simulink library "sm_trackV_lib_belt_underc_idlerArm_i2u0l3"  (R2026a)
settings: Solver=VariableStepAuto
undefined symbols (not defined in the file): A, Fixed, L1, L2, L3, Right, S, Trac, X, Y, Z
libraries: sm_lib x11, sm_trackV_lib_belt_underc_elem x9, nesl_utility x7, fl_lib x2, sm_trackV_lib_frame_idlerArm_i2u0l3 x1
(part 2 of 2)

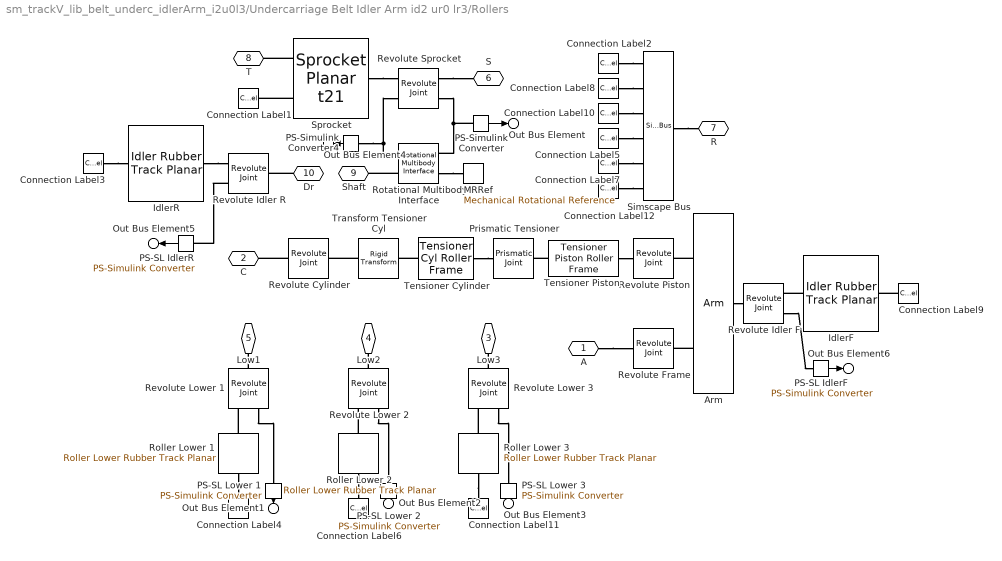
== system sm_trackV_lib_belt_underc_idlerArm_i2u0l3/Undercarriage Belt Idler Arm id2 ur0 lr3/Rollers ==
  Arm : sm_trackV_lib_belt_underc_elem/Arm  arm_idlerc=arm_idlerc  arm_tens_x=arm_tens_x  arm_tens_y=arm_tens_y  arm_wid=arm_wid  arm_thk=arm_thk  arm_rho=arm_rho  arm_clr=arm_clr  arm_opc=arm_opc
  Connection Label1 : ConnectionLabel  Label=S
  Connection Label10 : ConnectionLabel  Label=A
  Connection Label11 : ConnectionLabel  Label=L3
  Connection Label12 : ConnectionLabel  Label=L3
  Connection Label2 : ConnectionLabel  Label=S
  Connection Label3 : ConnectionLabel  Label=X
  Connection Label4 : ConnectionLabel  Label=L1
  Connection Label5 : ConnectionLabel  Label=L1
  Connection Label6 : ConnectionLabel  Label=L2
  Connection Label7 : ConnectionLabel  Label=L2
  Connection Label8 : ConnectionLabel  Label=X
  Connection Label9 : ConnectionLabel  Label=A
  IdlerF : sm_trackV_lib_belt_underc_elem/Idler Rubber Track Planar  idler_rad=idlerF_rad  idler_len=idlerF_len  wheel_clr=idlerF_wheel_clr  rim_rad=IdlerF_rim_rad  rim_hub_rad=idlerF_rim_hub_rad  rim_xc=idlerF_rim_xc  idler_rho=idlerF_rho  idler_opc=idlerF_opc  idler_clr=idlerF_clr  idler_axle_rad=idlerF_axle_rad  idler_axle_len=idlerF_axle_len  idler_axle_rho=idlerF_axle_rho  idler_axle_opc=idlerF_axle_opc  idler_axle_clr=idlerF_axle_clr  idler_contgeo_clr=idlerF_contgeo_clr  idler_contgeo_opc=idlerF_contgeo_opc
  IdlerR : sm_trackV_lib_belt_underc_elem/Idler Rubber Track Planar  idler_rad=idlerR_rad  idler_len=idlerR_len  wheel_clr=idlerR_wheel_clr  rim_rad=idlerR_rim_rad  rim_hub_rad=idlerR_rim_hub_rad  rim_xc=idlerR_rim_xc  idler_rho=idlerR_rho  idler_opc=idlerR_opc  idler_clr=idlerR_clr  idler_axle_rad=idlerR_axle_rad  idler_axle_len=idlerR_axle_len  idler_axle_rho=idlerR_axle_rho  idler_axle_opc=idlerR_axle_opc  idler_axle_clr=idlerR_axle_clr  idler_contgeo_clr=idlerR_contgeo_clr  idler_contgeo_opc=idlerR_contgeo_opc
  MRRef : fl_lib/Mechanical/Rotational Elements/Mechanical Rotational Reference
  PS-SL IdlerF : nesl_utility/PS-Simulink Converter  PhysicalDomain=network_engine_domain  SubClassName=ps_output  LeftPortType=input  RightPortType=output  PseudoPeriodic=off  Frequencies=[]  VectorFormat=inherit  Unit=inherit  AffineConversion=off
  PS-SL IdlerR : nesl_utility/PS-Simulink Converter  PhysicalDomain=network_engine_domain  SubClassName=ps_output  LeftPortType=input  RightPortType=output  PseudoPeriodic=off  Frequencies=[]  VectorFormat=inherit  Unit=inherit  AffineConversion=off
  PS-SL Lower 1 : nesl_utility/PS-Simulink Converter  PhysicalDomain=network_engine_domain  SubClassName=ps_output  LeftPortType=input  RightPortType=output  PseudoPeriodic=off  Frequencies=[]  VectorFormat=inherit  Unit=inherit  AffineConversion=off
  PS-SL Lower 2 : nesl_utility/PS-Simulink Converter  PhysicalDomain=network_engine_domain  SubClassName=ps_output  LeftPortType=input  RightPortType=output  PseudoPeriodic=off  Frequencies=[]  VectorFormat=inherit  Unit=inherit  AffineConversion=off
  PS-SL Lower 3 : nesl_utility/PS-Simulink Converter  PhysicalDomain=network_engine_domain  SubClassName=ps_output  LeftPortType=input  RightPortType=output  PseudoPeriodic=off  Frequencies=[]  VectorFormat=inherit  Unit=inherit  AffineConversion=off
  PS-Simulink Converter : nesl_utility/PS-Simulink Converter  PhysicalDomain=network_engine_domain  SubClassName=ps_output  LeftPortType=input  RightPortType=output  PseudoPeriodic=off  Frequencies=[]  VectorFormat=inherit  Unit=inherit  AffineConversion=off
  PS-Simulink Converter4 : nesl_utility/PS-Simulink Converter  PhysicalDomain=network_engine_domain  SubClassName=ps_output  LeftPortType=input  RightPortType=output  PseudoPeriodic=off  Frequencies=[]  VectorFormat=inherit  Unit=inherit  AffineConversion=off
  Prismatic Tensioner : sm_lib/Joints/Prismatic Joint  JointMode=Normal  CompositeWrenchDir=FollowerOnBase  CompositeWrenchFrame=BaseFrame  SenseConstraintForce=off  SenseConstraintTorque=off  SenseTotalForce=off  SenseTotalTorque=off  PositionTargetSpecify=on  PositionTargetPriority=High  PositionTargetValue=tensioner_x0  PositionTargetValueUnits=m  VelocityTargetSpecify=off  VelocityTargetPriority=High  VelocityTargetValue=0  VelocityTargetValueUnits=m/s  EquilibriumPosition=tensioner_eqpos  EquilibriumPositionUnits=m  SpringStiffness=tensioner_k  SpringStiffnessUnits=N/m  DampingCoefficient=tensioner_b  DampingCoefficientUnits=N/(m/s)  LowerLimitSpecify=off  LowerLimitBound=-1  LowerLimitBoundUnits=m  LowerLimitStiffness=1e6  LowerLimitStiffnessUnits=N/m  LowerLimitDamping=1e3  LowerLimitDampingUnits=N/(m/s)  LowerLimitTransitionRegionWidth=1e-4  LowerLimitTransitionRegionWidthUnits=m  UpperLimitSpecify=off  UpperLimitBound=1  UpperLimitBoundUnits=m  UpperLimitStiffness=1e6  UpperLimitStiffnessUnits=N/m  UpperLimitDamping=1e3  UpperLimitDampingUnits=N/(m/s)  UpperLimitTransitionRegionWidth=1e-4  UpperLimitTransitionRegionWidthUnits=m  TorqueActuationMode=NoTorque  MotionActuationMode=ComputedMotion  SensePosition=off  SenseVelocity=off  SenseAcceleration=off  SenseTorqueForce=off  SenseLowerLimitTorqueForce=off  SenseUpperLimitTorqueForce=off
  Revolute Cylinder : sm_lib/Joints/Revolute Joint  JointMode=Normal  CompositeWrenchDir=FollowerOnBase  CompositeWrenchFrame=BaseFrame  SenseConstraintForce=off  SenseConstraintTorque=off  SenseTotalForce=off  SenseTotalTorque=off  PositionTargetSpecify=on  PositionTargetPriority=Low  PositionTargetValue=0  PositionTargetValueUnits=deg  VelocityTargetSpecify=off  VelocityTargetPriority=High  VelocityTargetValue=0  VelocityTargetValueUnits=deg/s  EquilibriumPosition=0  EquilibriumPositionUnits=deg  SpringStiffness=0  SpringStiffnessUnits=N*m/deg  DampingCoefficient=0  DampingCoefficientUnits=N*m/(deg/s)  LowerLimitSpecify=off  LowerLimitBound=-90  LowerLimitBoundUnits=deg  LowerLimitStiffness=1e4  LowerLimitStiffnessUnits=N*m/deg  LowerLimitDamping=10  LowerLimitDampingUnits=N*m/(deg/s)  LowerLimitTransitionRegionWidth=0.1  LowerLimitTransitionRegionWidthUnits=deg  UpperLimitSpecify=off  UpperLimitBound=90  UpperLimitBoundUnits=deg  UpperLimitStiffness=1e4  UpperLimitStiffnessUnits=N*m/deg  UpperLimitDamping=10  UpperLimitDampingUnits=N*m/(deg/s)  UpperLimitTransitionRegionWidth=0.1  UpperLimitTransitionRegionWidthUnits=deg  TorqueActuationMode=NoTorque  MotionActuationMode=ComputedMotion  SensePosition=off  SenseVelocity=off  SenseAcceleration=off  SenseTorqueForce=off  SenseLowerLimitTorqueForce=off  SenseUpperLimitTorqueForce=off
  Revolute Frame : sm_lib/Joints/Revolute Joint  JointMode=Normal  CompositeWrenchDir=FollowerOnBase  CompositeWrenchFrame=BaseFrame  SenseConstraintForce=off  SenseConstraintTorque=off  SenseTotalForce=off  SenseTotalTorque=off  PositionTargetSpecify=off  PositionTargetPriority=Low  PositionTargetValue=0  PositionTargetValueUnits=deg  VelocityTargetSpecify=off  VelocityTargetPriority=High  VelocityTargetValue=0  VelocityTargetValueUnits=deg/s  EquilibriumPosition=0  EquilibriumPositionUnits=rad  SpringStiffness=0  SpringStiffnessUnits=N*m/rad  DampingCoefficient=0  DampingCoefficientUnits=N*m/(rad/s)  LowerLimitSpecify=off  LowerLimitBound=-90  LowerLimitBoundUnits=deg  LowerLimitStiffness=1e4  LowerLimitStiffnessUnits=N*m/deg  LowerLimitDamping=10  LowerLimitDampingUnits=N*m/(deg/s)  LowerLimitTransitionRegionWidth=0.1  LowerLimitTransitionRegionWidthUnits=deg  UpperLimitSpecify=off  UpperLimitBound=90  UpperLimitBoundUnits=deg  UpperLimitStiffness=1e4  UpperLimitStiffnessUnits=N*m/deg  UpperLimitDamping=10  UpperLimitDampingUnits=N*m/(deg/s)  UpperLimitTransitionRegionWidth=0.1  UpperLimitTransitionRegionWidthUnits=deg  TorqueActuationMode=NoTorque  MotionActuationMode=ComputedMotion  SensePosition=off  SenseVelocity=off  SenseAcceleration=off  SenseTorqueForce=off  SenseLowerLimitTorqueForce=off  SenseUpperLimitTorqueForce=off
  Revolute Idler F : sm_lib/Joints/Revolute Joint  JointMode=Normal  CompositeWrenchDir=FollowerOnBase  CompositeWrenchFrame=BaseFrame  SenseConstraintForce=on  SenseConstraintTorque=off  SenseTotalForce=off  SenseTotalTorque=off  PositionTargetSpecify=off  PositionTargetPriority=Low  PositionTargetValue=0  PositionTargetValueUnits=deg  VelocityTargetSpecify=off  VelocityTargetPriority=High  VelocityTargetValue=0  VelocityTargetValueUnits=deg/s  EquilibriumPosition=0  EquilibriumPositionUnits=rad  SpringStiffness=0  SpringStiffnessUnits=N*m/rad  DampingCoefficient=0  DampingCoefficientUnits=N*m/(rad/s)  LowerLimitSpecify=off  LowerLimitBound=-90  LowerLimitBoundUnits=deg  LowerLimitStiffness=1e4  LowerLimitStiffnessUnits=N*m/deg  LowerLimitDamping=10  LowerLimitDampingUnits=N*m/(deg/s)  LowerLimitTransitionRegionWidth=0.1  LowerLimitTransitionRegionWidthUnits=deg  UpperLimitSpecify=off  UpperLimitBound=90  UpperLimitBoundUnits=deg  UpperLimitStiffness=1e4  UpperLimitStiffnessUnits=N*m/deg  UpperLimitDamping=10  UpperLimitDampingUnits=N*m/(deg/s)  UpperLimitTransitionRegionWidth=0.1  UpperLimitTransitionRegionWidthUnits=deg  TorqueActuationMode=NoTorque  MotionActuationMode=ComputedMotion  SensePosition=off  SenseVelocity=off  SenseAcceleration=off  SenseTorqueForce=off  SenseLowerLimitTorqueForce=off  SenseUpperLimitTorqueForce=off
  Revolute Idler R : sm_lib/Joints/Revolute Joint  JointMode=Normal  CompositeWrenchDir=FollowerOnBase  CompositeWrenchFrame=BaseFrame  SenseConstraintForce=on  SenseConstraintTorque=off  SenseTotalForce=off  SenseTotalTorque=off  PositionTargetSpecify=off  PositionTargetPriority=Low  PositionTargetValue=0  PositionTargetValueUnits=deg  VelocityTargetSpecify=off  VelocityTargetPriority=High  VelocityTargetValue=0  VelocityTargetValueUnits=deg/s  EquilibriumPosition=0  EquilibriumPositionUnits=rad  SpringStiffness=0  SpringStiffnessUnits=N*m/rad  DampingCoefficient=0  DampingCoefficientUnits=N*m/(rad/s)  LowerLimitSpecify=off  LowerLimitBound=-90  LowerLimitBoundUnits=deg  LowerLimitStiffness=1e4  LowerLimitStiffnessUnits=N*m/deg  LowerLimitDamping=10  LowerLimitDampingUnits=N*m/(deg/s)  LowerLimitTransitionRegionWidth=0.1  LowerLimitTransitionRegionWidthUnits=deg  UpperLimitSpecify=off  UpperLimitBound=90  UpperLimitBoundUnits=deg  UpperLimitStiffness=1e4  UpperLimitStiffnessUnits=N*m/deg  UpperLimitDamping=10  UpperLimitDampingUnits=N*m/(deg/s)  UpperLimitTransitionRegionWidth=0.1  UpperLimitTransitionRegionWidthUnits=deg  TorqueActuationMode=NoTorque  MotionActuationMode=ComputedMotion  SensePosition=off  SenseVelocity=off  SenseAcceleration=off  SenseTorqueForce=off  SenseLowerLimitTorqueForce=off  SenseUpperLimitTorqueForce=off
  Revolute Lower 1 : sm_lib/Joints/Revolute Joint  JointMode=Normal  CompositeWrenchDir=FollowerOnBase  CompositeWrenchFrame=BaseFrame  SenseConstraintForce=on  SenseConstraintTorque=off  SenseTotalForce=off  SenseTotalTorque=off  PositionTargetSpecify=off  PositionTargetPriority=Low  PositionTargetValue=0  PositionTargetValueUnits=deg  VelocityTargetSpecify=off  VelocityTargetPriority=High  VelocityTargetValue=0  VelocityTargetValueUnits=deg/s  EquilibriumPosition=0  EquilibriumPositionUnits=rad  SpringStiffness=0  SpringStiffnessUnits=N*m/rad  DampingCoefficient=0  DampingCoefficientUnits=N*m/(rad/s)  LowerLimitSpecify=off  LowerLimitBound=-90  LowerLimitBoundUnits=deg  LowerLimitStiffness=1e4  LowerLimitStiffnessUnits=N*m/deg  LowerLimitDamping=10  LowerLimitDampingUnits=N*m/(deg/s)  LowerLimitTransitionRegionWidth=0.1  LowerLimitTransitionRegionWidthUnits=deg  UpperLimitSpecify=off  UpperLimitBound=90  UpperLimitBoundUnits=deg  UpperLimitStiffness=1e4  UpperLimitStiffnessUnits=N*m/deg  UpperLimitDamping=10  UpperLimitDampingUnits=N*m/(deg/s)  UpperLimitTransitionRegionWidth=0.1  UpperLimitTransitionRegionWidthUnits=deg  TorqueActuationMode=NoTorque  MotionActuationMode=ComputedMotion  SensePosition=off  SenseVelocity=off  SenseAcceleration=off  SenseTorqueForce=off  SenseLowerLimitTorqueForce=off  SenseUpperLimitTorqueForce=off
  Revolute Lower 2 : sm_lib/Joints/Revolute Joint  JointMode=Normal  CompositeWrenchDir=FollowerOnBase  CompositeWrenchFrame=BaseFrame  SenseConstraintForce=on  SenseConstraintTorque=off  SenseTotalForce=off  SenseTotalTorque=off  PositionTargetSpecify=off  PositionTargetPriority=Low  PositionTargetValue=0  PositionTargetValueUnits=deg  VelocityTargetSpecify=off  VelocityTargetPriority=High  VelocityTargetValue=0  VelocityTargetValueUnits=deg/s  EquilibriumPosition=0  EquilibriumPositionUnits=rad  SpringStiffness=0  SpringStiffnessUnits=N*m/rad  DampingCoefficient=0  DampingCoefficientUnits=N*m/(rad/s)  LowerLimitSpecify=off  LowerLimitBound=-90  LowerLimitBoundUnits=deg  LowerLimitStiffness=1e4  LowerLimitStiffnessUnits=N*m/deg  LowerLimitDamping=10  LowerLimitDampingUnits=N*m/(deg/s)  LowerLimitTransitionRegionWidth=0.1  LowerLimitTransitionRegionWidthUnits=deg  UpperLimitSpecify=off  UpperLimitBound=90  UpperLimitBoundUnits=deg  UpperLimitStiffness=1e4  UpperLimitStiffnessUnits=N*m/deg  UpperLimitDamping=10  UpperLimitDampingUnits=N*m/(deg/s)  UpperLimitTransitionRegionWidth=0.1  UpperLimitTransitionRegionWidthUnits=deg  TorqueActuationMode=NoTorque  MotionActuationMode=ComputedMotion  SensePosition=off  SenseVelocity=off  SenseAcceleration=off  SenseTorqueForce=off  SenseLowerLimitTorqueForce=off  SenseUpperLimitTorqueForce=off
  Revolute Lower 3 : sm_lib/Joints/Revolute Joint  JointMode=Normal  CompositeWrenchDir=FollowerOnBase  CompositeWrenchFrame=BaseFrame  SenseConstraintForce=on  SenseConstraintTorque=off  SenseTotalForce=off  SenseTotalTorque=off  PositionTargetSpecify=off  PositionTargetPriority=Low  PositionTargetValue=0  PositionTargetValueUnits=deg  VelocityTargetSpecify=off  VelocityTargetPriority=High  VelocityTargetValue=0  VelocityTargetValueUnits=deg/s  EquilibriumPosition=0  EquilibriumPositionUnits=rad  SpringStiffness=0  SpringStiffnessUnits=N*m/rad  DampingCoefficient=0  DampingCoefficientUnits=N*m/(rad/s)  LowerLimitSpecify=off  LowerLimitBound=-90  LowerLimitBoundUnits=deg  LowerLimitStiffness=1e4  LowerLimitStiffnessUnits=N*m/deg  LowerLimitDamping=10  LowerLimitDampingUnits=N*m/(deg/s)  LowerLimitTransitionRegionWidth=0.1  LowerLimitTransitionRegionWidthUnits=deg  UpperLimitSpecify=off  UpperLimitBound=90  UpperLimitBoundUnits=deg  UpperLimitStiffness=1e4  UpperLimitStiffnessUnits=N*m/deg  UpperLimitDamping=10  UpperLimitDampingUnits=N*m/(deg/s)  UpperLimitTransitionRegionWidth=0.1  UpperLimitTransitionRegionWidthUnits=deg  TorqueActuationMode=NoTorque  MotionActuationMode=ComputedMotion  SensePosition=off  SenseVelocity=off  SenseAcceleration=off  SenseTorqueForce=off  SenseLowerLimitTorqueForce=off  SenseUpperLimitTorqueForce=off
  Revolute Piston : sm_lib/Joints/Revolute Joint  JointMode=Normal  CompositeWrenchDir=FollowerOnBase  CompositeWrenchFrame=BaseFrame  SenseConstraintForce=off  SenseConstraintTorque=off  SenseTotalForce=off  SenseTotalTorque=off  PositionTargetSpecify=off  PositionTargetPriority=Low  PositionTargetValue=0  PositionTargetValueUnits=deg  VelocityTargetSpecify=off  VelocityTargetPriority=High  VelocityTargetValue=0  VelocityTargetValueUnits=deg/s  EquilibriumPosition=0  EquilibriumPositionUnits=rad  SpringStiffness=0  SpringStiffnessUnits=N*m/rad  DampingCoefficient=0  DampingCoefficientUnits=N*m/(rad/s)  LowerLimitSpecify=off  LowerLimitBound=-90  LowerLimitBoundUnits=deg  LowerLimitStiffness=1e4  LowerLimitStiffnessUnits=N*m/deg  LowerLimitDamping=10  LowerLimitDampingUnits=N*m/(deg/s)  LowerLimitTransitionRegionWidth=0.1  LowerLimitTransitionRegionWidthUnits=deg  UpperLimitSpecify=off  UpperLimitBound=90  UpperLimitBoundUnits=deg  UpperLimitStiffness=1e4  UpperLimitStiffnessUnits=N*m/deg  UpperLimitDamping=10  UpperLimitDampingUnits=N*m/(deg/s)  UpperLimitTransitionRegionWidth=0.1  UpperLimitTransitionRegionWidthUnits=deg  TorqueActuationMode=NoTorque  MotionActuationMode=ComputedMotion  SensePosition=off  SenseVelocity=off  SenseAcceleration=off  SenseTorqueForce=off  SenseLowerLimitTorqueForce=off  SenseUpperLimitTorqueForce=off
  Revolute Sprocket : sm_lib/Joints/Revolute Joint  JointMode=Normal  CompositeWrenchDir=FollowerOnBase  CompositeWrenchFrame=BaseFrame  SenseConstraintForce=off  SenseConstraintTorque=off  SenseTotalForce=off  SenseTotalTorque=off  PositionTargetSpecify=off  PositionTargetPriority=Low  PositionTargetValue=0  PositionTargetValueUnits=deg  VelocityTargetSpecify=off  VelocityTargetPriority=High  VelocityTargetValue=0  VelocityTargetValueUnits=deg/s  EquilibriumPosition=0  EquilibriumPositionUnits=rad  SpringStiffness=0  SpringStiffnessUnits=N*m/rad  DampingCoefficient=0  DampingCoefficientUnits=N*m/(rad/s)  LowerLimitSpecify=off  LowerLimitBound=-90  LowerLimitBoundUnits=deg  LowerLimitStiffness=1e4  LowerLimitStiffnessUnits=N*m/deg  LowerLimitDamping=10  LowerLimitDampingUnits=N*m/(deg/s)  LowerLimitTransitionRegionWidth=0.1  LowerLimitTransitionRegionWidthUnits=deg  UpperLimitSpecify=off  UpperLimitBound=90  UpperLimitBoundUnits=deg  UpperLimitStiffness=1e4  UpperLimitStiffnessUnits=N*m/deg  UpperLimitDamping=10  UpperLimitDampingUnits=N*m/(deg/s)  UpperLimitTransitionRegionWidth=0.1  UpperLimitTransitionRegionWidthUnits=deg  TorqueActuationMode=InputTorque  MotionActuationMode=ComputedMotion  SensePosition=off  SenseVelocity=on  SenseAcceleration=off  SenseTorqueForce=off  SenseLowerLimitTorqueForce=off  SenseUpperLimitTorqueForce=off
  Roller Lower 1 : sm_trackV_lib_belt_underc_elem/Roller Lower Rubber Track Planar  roller_lower_rad=roller_lower_rad  roller_lower_len=roller_lower_len  roller_lower_rho=roller_lower_rho  roller_lower_clr=roller_lower_clr  roller_lower_opc=roller_lower_opc  roller_lower_rim_thk=roller_lower_rim_thk  roller_lower_rim_len=roller_lower_rim_len  roller_lower_axle_rad=roller_lower_axle_rad  roller_lower_axle_len=roller_lower_axle_len  roller_lower_axle_rho=roller_lower_axle_rho  roller_lower_axle_opc=roller_lower_axle_opc  roller_lower_axle_clr=roller_lower_axle_clr  roller_lower_contgeo_clr=roller_lower_contgeo_clr  roller_lower_contgeo_opc=roller_lower_contgeo_opc
  Roller Lower 2 : sm_trackV_lib_belt_underc_elem/Roller Lower Rubber Track Planar  roller_lower_rad=roller_lower_rad  roller_lower_len=roller_lower_len  roller_lower_rho=roller_lower_rho  roller_lower_clr=roller_lower_clr  roller_lower_opc=roller_lower_opc  roller_lower_rim_thk=roller_lower_rim_thk  roller_lower_rim_len=roller_lower_rim_len  roller_lower_axle_rad=roller_lower_axle_rad  roller_lower_axle_len=roller_lower_axle_len  roller_lower_axle_rho=roller_lower_axle_rho  roller_lower_axle_opc=roller_lower_axle_opc  roller_lower_axle_clr=roller_lower_axle_clr  roller_lower_contgeo_clr=roller_lower_contgeo_clr  roller_lower_contgeo_opc=roller_lower_contgeo_opc
  Roller Lower 3 : sm_trackV_lib_belt_underc_elem/Roller Lower Rubber Track Planar  roller_lower_rad=roller_lower_rad  roller_lower_len=roller_lower_len  roller_lower_rho=roller_lower_rho  roller_lower_clr=roller_lower_clr  roller_lower_opc=roller_lower_opc  roller_lower_rim_thk=roller_lower_rim_thk  roller_lower_rim_len=roller_lower_rim_len  roller_lower_axle_rad=roller_lower_axle_rad  roller_lower_axle_len=roller_lower_axle_len  roller_lower_axle_rho=roller_lower_axle_rho  roller_lower_axle_opc=roller_lower_axle_opc  roller_lower_axle_clr=roller_lower_axle_clr  roller_lower_contgeo_clr=roller_lower_contgeo_clr  roller_lower_contgeo_opc=roller_lower_contgeo_opc
  Rotational Multibody Interface : fl_lib/Mechanical/Multibody Interfaces/Rotational Multibody Interface
  Simscape Bus : SimscapeBus  HierarchyStrings=S;X;A;L1;L2;L3
  Sprocket : sm_trackV_lib_belt_underc_elem/Sprocket Planar t21  sprk_wid_roll=sprk_wid_roll  sprk_rad_roll=sprk_rad_roll  sprk_opc=sprk_opc  sprk_clr=sprk_clr  sprk_rad_pitch=sprk_rad_pitch  sprk_spoke_rad=sprk_spoke_rad  sprk_spoke_len=sprk_spoke_len  sprk_spoke_num=sprk_spoke_num  sprk_spoke_clr=sprk_clr  sprk_spoke_opc=sprk_opc  rim_spoke_xc=sprk_rim_spoke_xc  rim_thk=sprk_rim_thk  rim_ir=sprk_rim_ir  sprk_contgeo_roller_clr=sprk_contgeo_roller_clr  sprk_contgeo_roller_opc=sprk_contgeo_roller_opc  sprk_contgeo_spoke_clr=sprk_contgeo_spoke_clr  sprk_contgeo_spoke_opc=sprk_contgeo_spoke_opc
  Tensioner Cylinder : sm_trackV_lib_belt_underc_elem/Tensioner Cyl Roller Frame  cyl_rad=tensioner_cyl_rad  cyl_len=tensioner_cyl_len  cyl_rho=tensioner_cyl_rho  cyl_clr=tensioner_cyl_clr  cyl_opc=tensioner_cyl_opc
  Tensioner Piston : sm_trackV_lib_belt_underc_elem/Tensioner Piston Roller Frame  pist_rad=tensioner_pist_rad  pist_len=pist_len  pist_rho=tensioner_pist_rho  pist_clr=tensioner_pist_clr  pist_opc=tensioner_pist_opc  br_height=tensioner_br_height  br_length=brk_len  br_width=tensioner_br_width  br_rho=tensioner_br_rho  br_thk=brk_thk  br_clr=tensioner_br_clr  br_opc=tensioner_br_opc
  Transform Tensioner Cyl : sm_lib/Frames and Transforms/Rigid Transform  RotationMethod=AlignedAxes  FollAlignAxisA=+Z  BaseAlignAxisA=+X  FollAlignAxisB=+X  BaseAlignAxisB=+Y  RotationStandardAxis=+Y  RotationAngle=90  RotationAngleUnits=deg  RotationArbitraryAxis=[0 0 1]  RotationSequenceAxes=FollowerAxes  RotationSequence=XYX  RotationSequenceAngles=[0 0 0]  RotationSequenceAnglesUnits=deg  RotationMatrix=[1 0 0; 0 1 0; 0 0 1]  Quaternion=[1 0 0 0]  TranslationMethod=None  TranslationCartesianOffset=[0 0 0]  TranslationCartesianOffsetUnits=m  TranslationStandardAxis=+Z  TranslationStandardOffset=0  TranslationStandardOffsetUnits=m  TranslationROffset=0  TranslationROffsetUnits=m  TranslationThetaOffset=0  TranslationThetaOffsetUnits=deg  TranslationZOffset=0  TranslationZOffsetUnits=m
  A : PMIOPort  Side=Left
  C : PMIOPort  Port=2  Side=Left
  Low3 : PMIOPort  Port=3  Side=Left
  Low2 : PMIOPort  Port=4  Side=Left
  Low1 : PMIOPort  Port=5  Side=Left
  S : PMIOPort  Port=6  Side=Left
  R : PMIOPort  Port=7  Side=Right
  T : PMIOPort  Port=8  Side=Right
  Shaft : PMIOPort  Port=9  Side=Right
  Dr : PMIOPort  Port=10  Side=Left
  Out Bus Element : Outport  PortName=m  Element=tSprk
  Out Bus Element1 : Outport  PortName=m  Element=RL1
  Out Bus Element2 : Outport  PortName=m  Element=RL2
  Out Bus Element3 : Outport  PortName=m  Element=RL3
  Out Bus Element4 : Outport  PortName=m  Element=wSprk
  Out Bus Element5 : Outport  PortName=m  Element=XIdlerR
  Out Bus Element6 : Outport  PortName=m  Element=XIdlerF
  wires:
  PS-Simulink Converter/1 -> Out Bus Element/1
  PS-SL Lower 1/1 -> Out Bus Element1/1
  PS-SL Lower 2/1 -> Out Bus Element2/1
  PS-SL Lower 3/1 -> Out Bus Element3/1
  PS-Simulink Converter4/1 -> Out Bus Element4/1
  PS-SL IdlerR/1 -> Out Bus Element5/1
  PS-SL IdlerF/1 -> Out Bus Element6/1
  connections:
  A/RConn1 -- Revolute Frame/LConn1
  Arm/LConn2 -- Revolute Frame/RConn1
  Tensioner Piston/RConn1 -- Revolute Piston/LConn1
  Arm/LConn1 -- Revolute Piston/RConn1
  Arm/RConn1 -- Revolute Idler F/LConn1
  Connection Label9/LConn1 -- IdlerF/RConn1
  Roller Lower 2/RConn1 -- Connection Label6/LConn1
  Revolute Sprocket/LConn1 -- S/RConn1
  Simscape Bus/RConn1 -- R/RConn1
  IdlerF/LConn1 -- Revolute Idler F/RConn1
  Sprocket/RConn1 -- Revolute Sprocket/RConn1
  Tensioner Cylinder/RConn1 -- Prismatic Tensioner/LConn1
  Revolute Lower 2/LConn1 -- Low2/RConn1
  Sprocket/LConn1 -- T/RConn1
  Roller Lower 1/RConn1 -- Connection Label4/LConn1
  Revolute Lower 1/LConn1 -- Low1/RConn1
  Connection Label8/LConn1 -- Simscape Bus/LConn2
  Connection Label2/LConn1 -- Simscape Bus/LConn1
  Tensioner Cylinder/LConn1 -- Transform Tensioner Cyl/RConn1
  Tensioner Piston/LConn1 -- Prismatic Tensioner/RConn1
  Roller Lower 2/LConn1 -- Revolute Lower 2/RConn1
  Roller Lower 1/LConn1 -- Revolute Lower 1/RConn1
  Revolute Sprocket/LConn2 -- Rotational Multibody Interface/LConn1 -- PS-Simulink Converter/LConn1
  Rotational Multibody Interface/RConn1 -- PS-Simulink Converter4/LConn1 -- Revolute Sprocket/RConn2
  Rotational Multibody Interface/RConn2 -- Shaft/RConn1
  Rotational Multibody Interface/LConn2 -- MRRef/LConn1
  IdlerR/LConn1 -- Revolute Idler R/RConn1
  Dr/RConn1 -- Revolute Idler R/LConn1
  Transform Tensioner Cyl/LConn1 -- Revolute Cylinder/RConn1
  Revolute Cylinder/LConn1 -- C/RConn1
  Sprocket/LConn2 -- Connection Label1/LConn1
  Connection Label10/LConn1 -- Simscape Bus/LConn3
  Connection Label3/LConn1 -- IdlerR/RConn1
  Connection Label5/LConn1 -- Simscape Bus/LConn4
  Connection Label7/LConn1 -- Simscape Bus/LConn5
  Roller Lower 3/LConn1 -- Revolute Lower 3/RConn1
  Revolute Lower 3/LConn1 -- Low3/RConn1
  Roller Lower 3/RConn1 -- Connection Label11/LConn1
  Connection Label12/LConn1 -- Simscape Bus/LConn6
  Revolute Lower 1/RConn2 -- PS-SL Lower 1/LConn1
  Revolute Lower 2/RConn2 -- PS-SL Lower 2/LConn1
  Revolute Lower 3/RConn2 -- PS-SL Lower 3/LConn1
  Revolute Idler R/RConn2 -- PS-SL IdlerR/LConn1
  Revolute Idler F/RConn2 -- PS-SL IdlerF/LConn1
